simulink model "AdaptiveCruiseControl_HapticInterface"  (R2022b)
settings: Solver=FixedStepDiscrete  StartTime=0.0  StopTime=10.0  FixedStep=0.0005  RelTol=1e-3  EnableMultiTasking=on
InitFcn:
  | mbd_s32k_consistency_checks(bdroot(gcs));
values from neighbouring files (symbols this model uses):
  Ak = 100    [parameters_template.m]
  b = 100    [parameters_template.m]
  base_ids = [10, 0, 0, 0, 0, 0]    [parameters_template.m]
  dT = 0.01    [parameters_template.m]
  H = 20    [parameters_template.m]
  Kd = 0.0358    [parameters_template.m]
  Kdm = 137.4    [parameters_template.m]
  Kp = 0.256    [parameters_template.m]
  Kpm = 573.45    [parameters_template.m]
  L1 = 1.6    [parameters_template.m]
  L2 = 0.8    [parameters_template.m]
  m = 2000    [parameters_template.m]
  n_desired = 0    [parameters_template.m]
  pot_gain = 0.8    [parameters_template.m]
  pot_offset = 512    [parameters_template.m]
  R = 1/5    (= 0.2)    [parameters_template.m]
  V_Ki = 50    [parameters_template.m]
  V_Kp = 5000    [parameters_template.m]
undefined symbols (not defined in the file or in its folder): DiscIntNeverNeededParam, LQFP
libraries: mbd_s32k1xx_ec_toolbox x38, slrealtimeutilitieslib x15, Veh_Sim x9, simulink x3
(part 2 of 2)

== system AdaptiveCruiseControl_HapticInterface/High Level Design/Outputs/Tx CAN ==
  note: Use pack block to generate data arrays
      | Do not use any mailbox buffers that are used for receives
  note: Use FCAN_Send block to transmit two messages to the CAN bus
  s,n,psi,us : Inport
  Byte Packing : slrealtimeutilitieslib/Byte Packing  MaskPackedDataType=uint8  MaskUnpackedDataTypes={'single','single'}  MaskAlignment=1
  Byte Packing1 : slrealtimeutilitieslib/Byte Packing  MaskPackedDataType=uint8  MaskUnpackedDataTypes={'single','single'}  MaskAlignment=1
  Constant : Constant  Value=8  OutDataTypeStr=uint8
  Constant1 : Constant  Value=8  OutDataTypeStr=uint8
  Demux : Demux
  FCAN_Send : mbd_s32k1xx_ec_toolbox/Communication Blocks/CAN Blocks/FCAN_Send  can_instance=0  can_mode=Non-blocking  can_timeout_ms=0  can_mb_idx=0  can_mb_init=On each call  show_id_input=off  can_extended_id=off  can_is_remote=off  can_id=4B  show_adv_opts=off  can_fd_enable=off  can_enable_brs=off  can_fd_padding=0
  FCAN_Send1 : mbd_s32k1xx_ec_toolbox/Communication Blocks/CAN Blocks/FCAN_Send  can_instance=0  can_mode=Non-blocking  can_timeout_ms=0  can_mb_idx=0  can_mb_init=On each call  show_id_input=off  can_extended_id=off  can_is_remote=off  can_id=4C  show_adv_opts=off  can_fd_enable=off  can_enable_brs=off  can_fd_padding=0
  wires:
  s,n,psi,us/1 -> Demux/1
  Demux/1 -> Byte Packing/1
  Demux/2 -> Byte Packing/2
  Byte Packing/1 -> FCAN_Send/1
  Constant/1 -> FCAN_Send/2
  Constant1/1 -> FCAN_Send1/2
  Byte Packing1/1 -> FCAN_Send1/1
  Demux/3 -> Byte Packing1/1
  Demux/4 -> Byte Packing1/2

== system AdaptiveCruiseControl_HapticInterface/High Level Design/Outputs/write torque ==
  Reaction Torque : Inport
  Constant : Constant  Value=0.5  OutDataTypeStr=double
  FTM_PWM_Config : mbd_s32k1xx_ec_toolbox/Motor Control Blocks/FTM Blocks/FTM_PWM_Config  ftmModule=0  ftmMode=Edge-Aligned PWM  ftmSourceClock=80 MHz  swcontrol_enable=off  chan0En=on  chan0Type=Complementary  chan2En=off  chan2Type=Independent  chan4En=off  chan4Type=Independent  chan6En=off  chan6Type=Independent  ftmPwmUnits=Hz  outFrequency=20000  ftmPeriod=4000  ftmPrescaler=Divide by 1  deadtimeUnits=Nanoseconds  deadtimeNs=0  deadtimeTicks=0  deadtimePrescaler=Divide by 1  dutyCycleCh0=0.25  dutyCycleCh1=0.25  dutyCycleCh2=0.25  dutyCycleCh3=0.25  dutyCycleCh4=0.25  dutyCycleCh5=0.25  dutyCycleCh6=0.25  dutyCycleCh7=0.25  dutyCycleSim=on  startAfterInit=on  showAdvOpt=on  pinFtmCh0=PTB12: [FTM0_CH0 | FTM Channel]  pinFtmCh1=None  pinPolCh0=Active High  pinPolCh1=Active Low  outputComplem0=Main duplicated  outputLevel0=Low  outputLevel1=Low  pinFtmCh2=PTC2: [FTM0_CH2 | FTM Channel]  pinFtmCh3=None  pinPolCh2=Active Low  pinPolCh3=Active Low  outputComplem2=Main duplicated  outputLevel2=Low  outputLevel3=Low  pinFtmCh4=PTB4: [FTM0_CH4 | FTM Channel]  pinFtmCh5=None  pinPolCh4=Active Low  pinPolCh5=Active Low  outputComplem4=Main duplicated  outputLevel4=Low  outputLevel5=Low  pinFtmCh6=PTA17: [FTM0_CH6 | FTM Channel]  pinFtmCh7=None  pinPolCh6=Active Low  pinPolCh7=Active Low  outputComplem6=Main duplicated  outputLevel6=Low  outputLevel7=Low  initTrigger=off  chTrigger0=off  chTrigger1=off  chTrigger2=off  chTrigger3=off  chTrigger4=off  chTrigger5=off  chTrigger6=off  chTrigger7=off  mcuTargetUpdate=on  pwmSyncTrg=Software trigger  pwmSyncHwRouting=TRGMUX_FTM7  pwmSyncTrg0=off  pwmSyncTrg1=off  pwmSyncTrg2=off  pwmSyncAutoClear=on  pwmSyncMinLoad=on  pwmSyncMaxLoad=on  pwmSyncInvert=System Clock  pwmSyncOutControl=System Clock  pwmSyncOutMask=System Clock  pwmSyncCounterInitial=System Clock  pwmSyncPoints=Update now  reloadEnable=off  reloadPriority=15  reloadHalfCycle=off  reloadHCR=0  reloadFrequency=0  chnMatch0=off  chnMatch1=off  chnMatch2=off  chnMatch3=off  chnMatch4=off  chnMatch5=off  chnMatch6=off  chnMatch7=off  pwmFaultProtection=off  pwmFaultInterrupt=off  pwmFaultClearing=Fault control disabled  pwmFaultPinState=Safe Value  pwmFaultFilterValue=0  pwmFaultPriority=15  fault_disen_0=off  fault_filter_0=off  fault_polarity_0=Active High  fault_disen_1=off  fault_filter_1=off  fault_polarity_1=Active high  fault_disen_2=off  fault_filter_2=off  fault_polarity_2=Active high  fault_disen_3=off  fault_filter_3=off  fault_polarity_3=Active high  fault_pin_0=None  fault_pin_1=None  fault_pin_2=None  fault_pin_3=None
  Gain : Gain  Gain=3.162e-4  OutDataTypeStr=single
  Saturation : Saturate  UpperLimit=0.76  LowerLimit=0.24
  Sum : Sum  Inputs=|++  OutDataTypeStr=single
  Terminator : Terminator
  wires:
  Saturation/1 -> FTM_PWM_Config/1
  Constant/1 -> Sum/2
  FTM_PWM_Config/1 -> Terminator/1
  Reaction Torque/1 -> Gain/1
  Gain/1 -> Sum/1
  Sum/1 -> Saturation/1

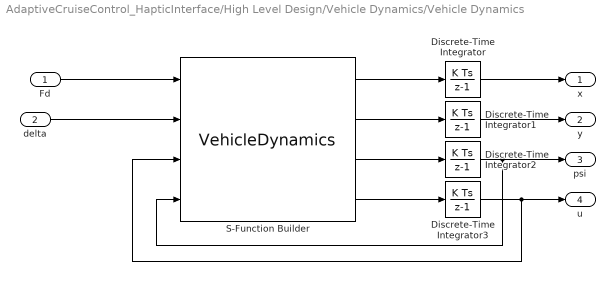
== system AdaptiveCruiseControl_HapticInterface/High Level Design/Vehicle Dynamics/Vehicle Dynamics ==
  Fd : Inport
  delta : Inport  Port=2
  Discrete-Time Integrator{,1..3} (4 alike) : DiscreteIntegrator  SampleTime=-1  ICPrevOutput=DiscIntNeverNeededParam  ICPrevScaledInput=DiscIntNeverNeededParam
  S-Function Builder : S-Function  FunctionName=VehicleDynamics  Parameters=L2,L1,b,m  SFunctionModules=VehicleDynamics_wrapper.c  SFunctionDeploymentMode=off  EnableBusSupport=off  mask(S-Function Builder){}
      mask help: Simulink:masks:SFunctionBuilder_MD
      mask init: same as AdaptiveCruiseControl_HapticInterface/High Level Design/ACC/Pick Lead Logic
      settings: CopyFcn=set_param(gcbh,'LinkStatus','none')  OpenFcn=sfunctionwizard(gcbh)
      mask Display:
      | plot(val(:,1),val(:,2))
      | disp(sys)
      | port_label('input',1,sprintf('%s', 'F\_d'),'interpreter','tex')
      | port_label('input',2,sprintf('%s', 'delta'),'interpreter','tex')
      | port_label('input',3,sprintf('%s', 'u'),'interpreter','tex')
      | port_label('input',4,sprintf('%s', 'psi'),'interpreter','tex')
      | port_label('output',1,sprintf('%s', 'x\_dot'),'interpreter','tex')
      | port_label('output',2,sprintf('%s', 'y\_dot'),'interpreter','tex')
      | port_label('output',3,sprintf('%s', 'psi\_dot'),'interpreter','tex')
      | port_label('output',4,sprintf('%s', 'u\_dot'),'interpreter','tex')
  x : Outport
  y : Outport  Port=2
  psi : Outport  Port=3
  u : Outport  Port=4
  wires:
  S-Function Builder/2 -> Discrete-Time Integrator1/1
  Discrete-Time Integrator2/1 -> S-Function Builder/4, psi/1
  S-Function Builder/3 -> Discrete-Time Integrator2/1
  S-Function Builder/1 -> Discrete-Time Integrator/1
  Discrete-Time Integrator/1 -> x/1
  S-Function Builder/4 -> Discrete-Time Integrator3/1
  Discrete-Time Integrator1/1 -> y/1
  Discrete-Time Integrator3/1 -> S-Function Builder/3, u/1
  delta/1 -> S-Function Builder/2
  Fd/1 -> S-Function Builder/1

== system AdaptiveCruiseControl_HapticInterface/High Level Design/Vehicle Dynamics/u_s calc ==
  s : Inport
  psi : Inport  Port=2
  u : Inport  Port=3
  delta : Inport  Port=4
  Look up Forward Vector : Veh_Sim/Look up Forward Vector  SystemSampleTime=-1  VariantActivationTime=update diagram  Latency=0  AutoFrameSizeCalculation=off
  S-Function Builder : S-Function  FunctionName=u_s_calc  SFunctionModules=u_s_calc_wrapper.c  SFunctionDeploymentMode=off  EnableBusSupport=off  mask(S-Function Builder){}
      mask help: Simulink:masks:SFunctionBuilder_MD
      mask init: same as AdaptiveCruiseControl_HapticInterface/High Level Design/ACC/Pick Lead Logic
      settings: CopyFcn=set_param(gcbh,'LinkStatus','none')  OpenFcn=sfunctionwizard(gcbh)
      mask Display:
      | plot(val(:,1),val(:,2))
      | disp(sys)
      | port_label('input',1,sprintf('%s', 'phi'),'interpreter','tex')
      | port_label('input',2,sprintf('%s', 'delta'),'interpreter','tex')
      | port_label('input',3,sprintf('%s', 'fx'),'interpreter','tex')
      | port_label('input',4,sprintf('%s', 'fy'),'interpreter','tex')
      | port_label('input',5,sprintf('%s', 'u'),'interpreter','tex')
      | port_label('output',1,sprintf('%s', 'u\_s'),'interpreter','tex')
  u_s : Outport
  wires:
  s/1 -> Look up Forward Vector/1
  u/1 -> S-Function Builder/5
  delta/1 -> S-Function Builder/2
  psi/1 -> S-Function Builder/1
  Look up Forward Vector/1 -> S-Function Builder/3
  Look up Forward Vector/2 -> S-Function Builder/4
  S-Function Builder/1 -> u_s/1

== system AdaptiveCruiseControl_HapticInterface/Serial Sim Out to Virtual Sim/UART Iteration/Resettable Subsystem ==
  Reset : ResetPort  DisableCoverage=on  ResetTriggerType=either
  Constant : Constant
  Delay : Delay  DelayLength=1
  Sum : Sum  Inputs=|++
  Out1 : Outport  VectorParamsAs1DForOutWhenUnconnected=off
  wires:
  Delay/1 -> Sum/1
  Constant/1 -> Sum/2
  Sum/1 -> Out1/1, Delay/1

== system AdaptiveCruiseControl_HapticInterface/Can Network Inputs/Extract CAN data/Data to s,n,psi,us /Switch Case Action Subsystem2 ==
  s,n : Inport
  Action Port : ActionPort  ActionPortLabel=if(u1 == 5)
  "Byte Unpacking " : slrealtimeutilitieslib/Byte Unpacking  MaskUnpackedDataTypes={'single', 'single'}  MaskUnpackedDataSizes={[1], [1]}  MaskAlignment=1
  s : Outport  VectorParamsAs1DForOutWhenUnconnected=off
  n : Outport  Port=2  VectorParamsAs1DForOutWhenUnconnected=off
  wires:
  s,n/1 -> "Byte Unpacking "/1
  "Byte Unpacking "/1 -> s/1
  "Byte Unpacking "/2 -> n/1

== system AdaptiveCruiseControl_HapticInterface/Can Network Inputs/Extract CAN data/Data to s,n,psi,us /Switch Case Action Subsystem3 ==
  psi,us : Inport
  Action Port : ActionPort  ActionPortLabel=elseif(u1 == 6)
  "Byte Unpacking " : slrealtimeutilitieslib/Byte Unpacking  MaskUnpackedDataTypes={'single', 'single'}  MaskUnpackedDataSizes={[1], [1]}  MaskAlignment=1
  psi : Outport  VectorParamsAs1DForOutWhenUnconnected=off
  us : Outport  Port=2  VectorParamsAs1DForOutWhenUnconnected=off
  wires:
  psi,us/1 -> "Byte Unpacking "/1
  "Byte Unpacking "/1 -> psi/1
  "Byte Unpacking "/2 -> us/1

== system AdaptiveCruiseControl_HapticInterface/Can Network Inputs/Extract CAN data/Data to s,n,psi,us 1/Switch Case Action Subsystem2 ==
  s,n : Inport
  Action Port : ActionPort  ActionPortLabel=if(u1 == 5)
  "Byte Unpacking " : slrealtimeutilitieslib/Byte Unpacking  MaskUnpackedDataTypes={'single', 'single'}  MaskUnpackedDataSizes={[1], [1]}  MaskAlignment=1
  s : Outport  VectorParamsAs1DForOutWhenUnconnected=off
  n : Outport  Port=2  VectorParamsAs1DForOutWhenUnconnected=off
  wires:
  s,n/1 -> "Byte Unpacking "/1
  "Byte Unpacking "/1 -> s/1
  "Byte Unpacking "/2 -> n/1

== system AdaptiveCruiseControl_HapticInterface/Can Network Inputs/Extract CAN data/Data to s,n,psi,us 1/Switch Case Action Subsystem3 ==
  psi,us : Inport
  Action Port : ActionPort  ActionPortLabel=elseif(u1 == 6)
  "Byte Unpacking " : slrealtimeutilitieslib/Byte Unpacking  MaskUnpackedDataTypes={'single', 'single'}  MaskUnpackedDataSizes={[1], [1]}  MaskAlignment=1
  psi : Outport  VectorParamsAs1DForOutWhenUnconnected=off
  us : Outport  Port=2  VectorParamsAs1DForOutWhenUnconnected=off
  wires:
  psi,us/1 -> "Byte Unpacking "/1
  "Byte Unpacking "/1 -> psi/1
  "Byte Unpacking "/2 -> us/1

== system AdaptiveCruiseControl_HapticInterface/Can Network Inputs/Extract CAN data/Data to s,n,psi,us 2/Switch Case Action Subsystem2 ==
  s,n : Inport
  Action Port : ActionPort  ActionPortLabel=if(u1 == 5)
  "Byte Unpacking " : slrealtimeutilitieslib/Byte Unpacking  MaskUnpackedDataTypes={'single', 'single'}  MaskUnpackedDataSizes={[1], [1]}  MaskAlignment=1
  s : Outport  VectorParamsAs1DForOutWhenUnconnected=off
  n : Outport  Port=2  VectorParamsAs1DForOutWhenUnconnected=off
  wires:
  s,n/1 -> "Byte Unpacking "/1
  "Byte Unpacking "/1 -> s/1
  "Byte Unpacking "/2 -> n/1

== system AdaptiveCruiseControl_HapticInterface/Can Network Inputs/Extract CAN data/Data to s,n,psi,us 2/Switch Case Action Subsystem3 ==
  psi,us : Inport
  Action Port : ActionPort  ActionPortLabel=elseif(u1 == 6)
  "Byte Unpacking " : slrealtimeutilitieslib/Byte Unpacking  MaskUnpackedDataTypes={'single', 'single'}  MaskUnpackedDataSizes={[1], [1]}  MaskAlignment=1
  psi : Outport  VectorParamsAs1DForOutWhenUnconnected=off
  us : Outport  Port=2  VectorParamsAs1DForOutWhenUnconnected=off
  wires:
  psi,us/1 -> "Byte Unpacking "/1
  "Byte Unpacking "/1 -> psi/1
  "Byte Unpacking "/2 -> us/1

== system AdaptiveCruiseControl_HapticInterface/Can Network Inputs/Extract CAN data/Data to s,n,psi,us 3/Switch Case Action Subsystem2 ==
  s,n : Inport
  Action Port : ActionPort  ActionPortLabel=if(u1 == 5)
  "Byte Unpacking " : slrealtimeutilitieslib/Byte Unpacking  MaskUnpackedDataTypes={'single', 'single'}  MaskUnpackedDataSizes={[1], [1]}  MaskAlignment=1
  s : Outport  VectorParamsAs1DForOutWhenUnconnected=off
  n : Outport  Port=2  VectorParamsAs1DForOutWhenUnconnected=off
  wires:
  s,n/1 -> "Byte Unpacking "/1
  "Byte Unpacking "/1 -> s/1
  "Byte Unpacking "/2 -> n/1

== system AdaptiveCruiseControl_HapticInterface/Can Network Inputs/Extract CAN data/Data to s,n,psi,us 3/Switch Case Action Subsystem3 ==
  psi,us : Inport
  Action Port : ActionPort  ActionPortLabel=elseif(u1 == 6)
  "Byte Unpacking " : slrealtimeutilitieslib/Byte Unpacking  MaskUnpackedDataTypes={'single', 'single'}  MaskUnpackedDataSizes={[1], [1]}  MaskAlignment=1
  psi : Outport  VectorParamsAs1DForOutWhenUnconnected=off
  us : Outport  Port=2  VectorParamsAs1DForOutWhenUnconnected=off
  wires:
  psi,us/1 -> "Byte Unpacking "/1
  "Byte Unpacking "/1 -> psi/1
  "Byte Unpacking "/2 -> us/1

== system AdaptiveCruiseControl_HapticInterface/Can Network Inputs/Extract CAN data/Data to s,n,psi,us 4/Switch Case Action Subsystem2 ==
  s,n : Inport
  Action Port : ActionPort  ActionPortLabel=if(u1 == 5)
  "Byte Unpacking " : slrealtimeutilitieslib/Byte Unpacking  MaskUnpackedDataTypes={'single', 'single'}  MaskUnpackedDataSizes={[1], [1]}  MaskAlignment=1
  s : Outport  VectorParamsAs1DForOutWhenUnconnected=off
  n : Outport  Port=2  VectorParamsAs1DForOutWhenUnconnected=off
  wires:
  s,n/1 -> "Byte Unpacking "/1
  "Byte Unpacking "/1 -> s/1
  "Byte Unpacking "/2 -> n/1

== system AdaptiveCruiseControl_HapticInterface/Can Network Inputs/Extract CAN data/Data to s,n,psi,us 4/Switch Case Action Subsystem3 ==
  psi,us : Inport
  Action Port : ActionPort  ActionPortLabel=elseif(u1 == 6)
  "Byte Unpacking " : slrealtimeutilitieslib/Byte Unpacking  MaskUnpackedDataTypes={'single', 'single'}  MaskUnpackedDataSizes={[1], [1]}  MaskAlignment=1
  psi : Outport  VectorParamsAs1DForOutWhenUnconnected=off
  us : Outport  Port=2  VectorParamsAs1DForOutWhenUnconnected=off
  wires:
  psi,us/1 -> "Byte Unpacking "/1
  "Byte Unpacking "/1 -> psi/1
  "Byte Unpacking "/2 -> us/1

== system AdaptiveCruiseControl_HapticInterface/Can Network Inputs/Extract CAN data/Data to s,n,psi,us 5/Switch Case Action Subsystem2 ==
  s,n : Inport
  Action Port : ActionPort  ActionPortLabel=if(u1 == 5)
  "Byte Unpacking " : slrealtimeutilitieslib/Byte Unpacking  MaskUnpackedDataTypes={'single', 'single'}  MaskUnpackedDataSizes={[1], [1]}  MaskAlignment=1
  s : Outport  VectorParamsAs1DForOutWhenUnconnected=off
  n : Outport  Port=2  VectorParamsAs1DForOutWhenUnconnected=off
  wires:
  s,n/1 -> "Byte Unpacking "/1
  "Byte Unpacking "/1 -> s/1
  "Byte Unpacking "/2 -> n/1

== system AdaptiveCruiseControl_HapticInterface/Can Network Inputs/Extract CAN data/Data to s,n,psi,us 5/Switch Case Action Subsystem3 ==
  psi,us : Inport
  Action Port : ActionPort  ActionPortLabel=elseif(u1 == 6)
  "Byte Unpacking " : slrealtimeutilitieslib/Byte Unpacking  MaskUnpackedDataTypes={'single', 'single'}  MaskUnpackedDataSizes={[1], [1]}  MaskAlignment=1
  psi : Outport  VectorParamsAs1DForOutWhenUnconnected=off
  us : Outport  Port=2  VectorParamsAs1DForOutWhenUnconnected=off
  wires:
  psi,us/1 -> "Byte Unpacking "/1
  "Byte Unpacking "/1 -> psi/1
  "Byte Unpacking "/2 -> us/1

== system AdaptiveCruiseControl_HapticInterface/High Level Design/ACC/Speed Ctrl/PI ==
  Error : Inport
  Gain : Gain  Gain=V_Ki  SaturateOnIntegerOverflow=on  OutDataTypeStr=Inherit: Same as input  ParamDataTypeStr=Inherit: Same as input
  Gain1 : Gain  Gain=V_Kp  SaturateOnIntegerOverflow=on  OutDataTypeStr=Inherit: Same as input  ParamDataTypeStr=Inherit: Same as input
  My Discrete Integrator : Subsystem
  Sum : Sum  Inputs=|++  SaturateOnIntegerOverflow=on
  U : Outport
  wires:
  Sum/1 -> U/1
  Error/1 -> Gain1/1, Gain/1
  Gain1/1 -> Sum/2
  My Discrete Integrator/1(X) -> Sum/1
  Gain/1 -> My Discrete Integrator/1(X_dot)

== system AdaptiveCruiseControl_HapticInterface/High Level Design/Auto Steer/Subsystem1/Inner Loop PD ==
  In1 : Inport
  Gain1 : Gain  Gain=1/dT
  Gain3 : Gain  Gain=Kpm
  Gain4 : Gain  Gain=Kdm
  Sum : Sum  Inputs=|+-
  Sum2 : Sum  Inputs=|++
  Unit Delay : UnitDelay  SampleTime=-1  HasFrameUpgradeWarning=on
  "Auto-steer torque, Nmm" : Outport
  wires:
  Sum2/1 -> "Auto-steer torque, Nmm"/1  "Auto-steer torque, Nmm"
  Gain4/1 -> Sum2/1
  Gain3/1 -> Sum2/2
  In1/1 -> Unit Delay/1, Sum/1, Gain3/1
  Sum/1 -> Gain1/1
  Unit Delay/1 -> Sum/2
  Gain1/1 -> Gain4/1

== system AdaptiveCruiseControl_HapticInterface/High Level Design/Auto Steer/Subsystem1/Outerloop PD ==
  In2 : Inport
  Gain1 : Gain  Gain=1/dT
  Gain4 : Gain  Gain=Kp
  Gain6 : Gain  Gain=Kd
  Sum : Sum  Inputs=|+-
  Sum2 : Sum  Inputs=|++
  Unit Delay : UnitDelay  SampleTime=-1  HasFrameUpgradeWarning=on
  delta : Outport
  wires:
  Sum/1 -> Gain1/1
  In2/1 -> Gain4/1, Unit Delay/1, Sum/1
  Gain4/1 -> Sum2/2
  Sum2/1 -> delta/1
  Gain1/1 -> Gain6/1
  Gain6/1 -> Sum2/1
  Unit Delay/1 -> Sum/2

== system AdaptiveCruiseControl_HapticInterface/High Level Design/Outputs/Extract x,y,psi (Cars 1 - 6)/Extract x,y,psi ==
  s,n,psi,us : Inport
  Demux : Demux
  Mux : Mux  Inputs=3
  Terminator : Terminator
  s,n to x,y : Veh_Sim/s,n to x,y  SystemSampleTime=-1  VariantActivationTime=update diagram  Latency=0  AutoFrameSizeCalculation=off
  x,y,psi : Outport  VectorParamsAs1DForOutWhenUnconnected=off
  wires:
  Demux/1 -> s,n to x,y/1
  Demux/2 -> s,n to x,y/2
  s,n,psi,us/1 -> Demux/1
  s,n to x,y/1 -> Mux/1
  s,n to x,y/2 -> Mux/2
  Demux/3 -> Mux/3
  Mux/1 -> x,y,psi/1
  Demux/4 -> Terminator/1

== system AdaptiveCruiseControl_HapticInterface/High Level Design/Outputs/Extract x,y,psi (Cars 1 - 6)/Extract x,y,psi1 ==
  s,n,psi,us : Inport
  Demux : Demux
  Mux : Mux  Inputs=3
  Terminator : Terminator
  s,n to x,y : Veh_Sim/s,n to x,y  SystemSampleTime=-1  VariantActivationTime=update diagram  Latency=0  AutoFrameSizeCalculation=off
  x,y,psi : Outport  VectorParamsAs1DForOutWhenUnconnected=off
  wires:
  Demux/1 -> s,n to x,y/1
  Demux/2 -> s,n to x,y/2
  s,n,psi,us/1 -> Demux/1
  s,n to x,y/1 -> Mux/1
  s,n to x,y/2 -> Mux/2
  Demux/3 -> Mux/3
  Mux/1 -> x,y,psi/1
  Demux/4 -> Terminator/1

== system AdaptiveCruiseControl_HapticInterface/High Level Design/Outputs/Extract x,y,psi (Cars 1 - 6)/Extract x,y,psi2 ==
  s,n,psi,us : Inport
  Demux : Demux
  Mux : Mux  Inputs=3
  Terminator : Terminator
  s,n to x,y : Veh_Sim/s,n to x,y  SystemSampleTime=-1  VariantActivationTime=update diagram  Latency=0  AutoFrameSizeCalculation=off
  x,y,psi : Outport  VectorParamsAs1DForOutWhenUnconnected=off
  wires:
  Demux/1 -> s,n to x,y/1
  Demux/2 -> s,n to x,y/2
  s,n,psi,us/1 -> Demux/1
  s,n to x,y/1 -> Mux/1
  s,n to x,y/2 -> Mux/2
  Demux/3 -> Mux/3
  Mux/1 -> x,y,psi/1
  Demux/4 -> Terminator/1

== system AdaptiveCruiseControl_HapticInterface/High Level Design/Outputs/Extract x,y,psi (Cars 1 - 6)/Extract x,y,psi3 ==
  s,n,psi,us : Inport
  Demux : Demux
  Mux : Mux  Inputs=3
  Terminator : Terminator
  s,n to x,y : Veh_Sim/s,n to x,y  SystemSampleTime=-1  VariantActivationTime=update diagram  Latency=0  AutoFrameSizeCalculation=off
  x,y,psi : Outport  VectorParamsAs1DForOutWhenUnconnected=off
  wires:
  Demux/1 -> s,n to x,y/1
  Demux/2 -> s,n to x,y/2
  s,n,psi,us/1 -> Demux/1
  s,n to x,y/1 -> Mux/1
  s,n to x,y/2 -> Mux/2
  Demux/3 -> Mux/3
  Mux/1 -> x,y,psi/1
  Demux/4 -> Terminator/1

== system AdaptiveCruiseControl_HapticInterface/High Level Design/Outputs/Extract x,y,psi (Cars 1 - 6)/Extract x,y,psi4 ==
  s,n,psi,us : Inport
  Demux : Demux
  Mux : Mux  Inputs=3
  Terminator : Terminator
  s,n to x,y : Veh_Sim/s,n to x,y  SystemSampleTime=-1  VariantActivationTime=update diagram  Latency=0  AutoFrameSizeCalculation=off
  x,y,psi : Outport  VectorParamsAs1DForOutWhenUnconnected=off
  wires:
  Demux/1 -> s,n to x,y/1
  Demux/2 -> s,n to x,y/2
  s,n,psi,us/1 -> Demux/1
  s,n to x,y/1 -> Mux/1
  s,n to x,y/2 -> Mux/2
  Demux/3 -> Mux/3
  Mux/1 -> x,y,psi/1
  Demux/4 -> Terminator/1

== system AdaptiveCruiseControl_HapticInterface/High Level Design/Outputs/Extract x,y,psi (Cars 1 - 6)/Extract x,y,psi5 ==
  s,n,psi,us : Inport
  Demux : Demux
  Mux : Mux  Inputs=3
  Terminator : Terminator
  s,n to x,y : Veh_Sim/s,n to x,y  SystemSampleTime=-1  VariantActivationTime=update diagram  Latency=0  AutoFrameSizeCalculation=off
  x,y,psi : Outport  VectorParamsAs1DForOutWhenUnconnected=off
  wires:
  Demux/1 -> s,n to x,y/1
  Demux/2 -> s,n to x,y/2
  s,n,psi,us/1 -> Demux/1
  s,n to x,y/1 -> Mux/1
  s,n to x,y/2 -> Mux/2
  Demux/3 -> Mux/3
  Mux/1 -> x,y,psi/1
  Demux/4 -> Terminator/1

== system AdaptiveCruiseControl_HapticInterface/High Level Design/ACC/Speed Ctrl/PI/My Discrete Integrator ==
  X_dot : Inport
  Gain : Gain  Gain=dT  SaturateOnIntegerOverflow=on  OutDataTypeStr=Inherit: Same as input  ParamDataTypeStr=Inherit: Same as input
  Sum : Sum  Inputs=|++  InputSameDT=on  SaturateOnIntegerOverflow=on  OutDataTypeStr=Inherit: Same as first input
  Unit Delay : UnitDelay  SampleTime=-1  HasFrameUpgradeWarning=on
  X : Outport
  wires:
  Gain/1 -> Sum/1
  X_dot/1 -> Gain/1
  Sum/1 -> Unit Delay/1
  Unit Delay/1 -> Sum/2, X/1
